simulink subsystem "Plant"  (R2022a)
settings: Solver=VariableStepAuto  StartTime=0.0  StopTime=10.0  RelTol=1e-3
settings Model: Creator=mmarq  LastModifiedBy=mmarq

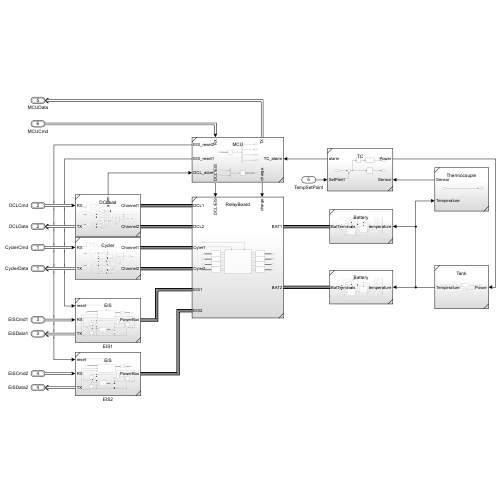
[thumbnail: Simulink's stored preview of the top-level diagram]
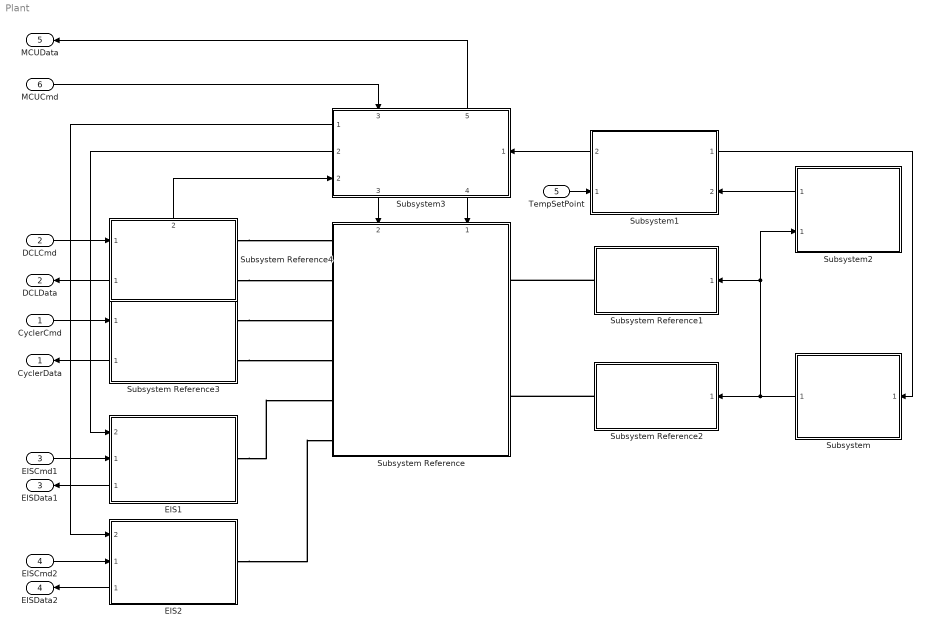
== system Plant ==
  CyclerCmd : Inport  OutputPortMessageModes=m  OutDataTypeStr=Bus: CyclerCmd  BusOutputAsStruct=on
  DCLCmd : Inport  OutputPortMessageModes=m  Port=2  OutDataTypeStr=Bus: DCLCmd  BusOutputAsStruct=on
  EISCmd1 : Inport  OutputPortMessageModes=m  Port=3  OutDataTypeStr=Bus: EISCmd  BusOutputAsStruct=on
  EISCmd2 : Inport  OutputPortMessageModes=m  Port=4  OutDataTypeStr=Bus: EISCmd  BusOutputAsStruct=on
  TempSetPoint : Inport  Port=5
  MCUCmd : Inport  OutputPortMessageModes=m  Port=6  OutDataTypeStr=Bus: MCUCmd  BusOutputAsStruct=on
  EIS1 : Subsystem  ReferencedSubsystem=EIS
      settings: PortSchema="{\"entries\":[{\"content\":{\"sides\":[{\"content\":{\"connectorIds\":[\"In2\",\"In1\",\"Out1\"]},\"type\":\"ConnectorPlacement.EquallySpacedRectSide\",\"uuid\":\"bda901de-5fc5-4df6-bed4-bf969933d972\"},{\"content\":{\"connectorIds\":[\"LConn1\"],\"side\":\"RIGHT\"},\"type\":\"ConnectorPlacement.EquallySpacedRectSide\",\"uuid\":\"97e6e5df-6a68-4cb9-aa40-ad9555eae5d3\"},{\"content\":{\"connectorIds\":[],\"side\":\"TOP\"},\"type\":\"ConnectorPlacement.EquallySpacedRectSide\",\"uuid\":\"3686a2fc-9119-406b-ac45-90d58aa6d823\"}]},\"type\":\"ConnectorPlacement.EquallySpacedConnector\",\"uuid\":\"6daecac9-5e0e-4dc6-b323-39bbe07465b3\"}],\"packageUris\":[\"http://schema.mathworks.com/mf0/Connector/R2020b\"],\"version\":\"1.0\"}"
  EIS2 : Subsystem  ReferencedSubsystem=EIS
      settings: PortSchema="{\"entries\":[{\"content\":{\"sides\":[{\"content\":{\"connectorIds\":[\"In2\",\"In1\",\"Out1\"]},\"type\":\"ConnectorPlacement.EquallySpacedRectSide\",\"uuid\":\"346fccca-2e03-4390-b8f8-dabc407f8e1d\"},{\"content\":{\"connectorIds\":[\"LConn1\"],\"side\":\"RIGHT\"},\"type\":\"ConnectorPlacement.EquallySpacedRectSide\",\"uuid\":\"347ef005-0f29-4770-89d9-3f34bb09e857\"},{\"content\":{\"connectorIds\":[],\"side\":\"TOP\"},\"type\":\"ConnectorPlacement.EquallySpacedRectSide\",\"uuid\":\"43d2187e-170b-4050-a904-0fbb5a542a24\"}]},\"type\":\"ConnectorPlacement.EquallySpacedConnector\",\"uuid\":\"0bc059c9-e074-4757-9a5e-e56a8190d977\"}],\"packageUris\":[\"http://schema.mathworks.com/mf0/Connector/R2020b\"],\"version\":\"1.0\"}"
  Subsystem : Subsystem  ReferencedSubsystem=Tank
  Subsystem Reference : Subsystem  ReferencedSubsystem=RelayBoard
      settings: PortSchema="{\"entries\":[{\"content\":{\"sides\":[{\"content\":{\"connectorIds\":[\"LConn3\",\"LConn7\",\"LConn2\",\"LConn6\",\"LConn4\",\"LConn8\"]},\"type\":\"ConnectorPlacement.EquallySpacedRectSide\",\"uuid\":\"2c82222c-b92b-4cb2-b168-0111504e6e71\"},{\"content\":{\"connectorIds\":[\"LConn1\",\"LConn5\"],\"side\":\"RIGHT\"},\"type\":\"ConnectorPlacement.EquallySpacedRectSide\",\"uuid\":\"59e2e9be-7ca9-4e66-8a31-f71f766dd2df\"},{\"content\":{\"connectorIds\":[\"In2\",\"In1\"],\"side\":\"TOP\"},\"type\":\"ConnectorPlacement.EquallySpacedRectSide\",\"uuid\":\"aebc3a48-61aa-4997-b1d8-73deb527f504\"}]},\"type\":\"ConnectorPlacement.EquallySpacedConnector\",\"uuid\":\"65ea92de-f703-4c73-ace1-0a27781508bc\"}],\"packageUris\":[\"http://schema.mathworks.com/mf0/Connector/R2020b\"],\"version\":\"1.0\"}"
  Subsystem Reference1 : Subsystem  ReferencedSubsystem=Battery
      settings: PortSchema="{\"entries\":[{\"content\":{\"sides\":[{\"content\":{\"connectorIds\":[\"LConn1\"]},\"type\":\"ConnectorPlacement.EquallySpacedRectSide\",\"uuid\":\"c15baa17-3528-45e3-b2fa-303e9d710e06\"},{\"content\":{\"connectorIds\":[\"In1\"],\"side\":\"RIGHT\"},\"type\":\"ConnectorPlacement.EquallySpacedRectSide\",\"uuid\":\"fb2fc25f-2319-470c-9cd2-01ed067f04f0\"},{\"content\":{\"connectorIds\":[],\"side\":\"TOP\"},\"type\":\"ConnectorPlacement.EquallySpacedRectSide\",\"uuid\":\"019a131c-ab68-4a32-933d-e5ce9d7fc5af\"}]},\"type\":\"ConnectorPlacement.EquallySpacedConnector\",\"uuid\":\"8ea13b11-84cd-4d75-b595-d58928f0c49e\"}],\"packageUris\":[\"http://schema.mathworks.com/mf0/Connector/R2020b\"],\"version\":\"1.0\"}"
  Subsystem Reference2 : Subsystem  ReferencedSubsystem=Battery
      settings: PortSchema="{\"entries\":[{\"content\":{\"sides\":[{\"content\":{\"connectorIds\":[\"LConn1\"]},\"type\":\"ConnectorPlacement.EquallySpacedRectSide\",\"uuid\":\"c15baa17-3528-45e3-b2fa-303e9d710e06\"},{\"content\":{\"connectorIds\":[\"In1\"],\"side\":\"RIGHT\"},\"type\":\"ConnectorPlacement.EquallySpacedRectSide\",\"uuid\":\"fb2fc25f-2319-470c-9cd2-01ed067f04f0\"},{\"content\":{\"connectorIds\":[],\"side\":\"TOP\"},\"type\":\"ConnectorPlacement.EquallySpacedRectSide\",\"uuid\":\"019a131c-ab68-4a32-933d-e5ce9d7fc5af\"}]},\"type\":\"ConnectorPlacement.EquallySpacedConnector\",\"uuid\":\"8ea13b11-84cd-4d75-b595-d58928f0c49e\"}],\"packageUris\":[\"http://schema.mathworks.com/mf0/Connector/R2020b\"],\"version\":\"1.0\"}"
  Subsystem Reference3 : Subsystem  ReferencedSubsystem=Cycler
      settings: PortSchema="{\"entries\":[{\"content\":{\"sides\":[{\"content\":{\"connectorIds\":[\"In1\",\"Out1\"]},\"type\":\"ConnectorPlacement.EquallySpacedRectSide\",\"uuid\":\"f71a85fa-5f1b-4f60-afc2-2af602cd6bfa\"},{\"content\":{\"connectorIds\":[\"LConn1\",\"LConn2\"],\"side\":\"RIGHT\"},\"type\":\"ConnectorPlacement.EquallySpacedRectSide\",\"uuid\":\"a58ae27e-7fda-4e3b-bf34-5bf7de7a0120\"},{\"content\":{\"connectorIds\":[],\"side\":\"TOP\"},\"type\":\"ConnectorPlacement.EquallySpacedRectSide\",\"uuid\":\"cf49a94a-a45d-4ba1-8d31-8fa348aa4236\"}]},\"type\":\"ConnectorPlacement.EquallySpacedConnector\",\"uuid\":\"5fb0b0ec-3310-4f5c-9c9c-9e0d49a0c2e5\"}],\"packageUris\":[\"http://schema.mathworks.com/mf0/Connector/R2020b\"],\"version\":\"1.0\"}"
  Subsystem Reference4 : Subsystem  ReferencedSubsystem=DCLoad
      settings: PortSchema="{\"entries\":[{\"content\":{\"sides\":[{\"content\":{\"connectorIds\":[\"In1\",\"Out1\"]},\"type\":\"ConnectorPlacement.EquallySpacedRectSide\",\"uuid\":\"f71a85fa-5f1b-4f60-afc2-2af602cd6bfa\"},{\"content\":{\"connectorIds\":[\"LConn1\",\"LConn2\"],\"side\":\"RIGHT\"},\"type\":\"ConnectorPlacement.EquallySpacedRectSide\",\"uuid\":\"a58ae27e-7fda-4e3b-bf34-5bf7de7a0120\"},{\"content\":{\"connectorIds\":[\"Out2\"],\"side\":\"TOP\"},\"type\":\"ConnectorPlacement.EquallySpacedRectSide\",\"uuid\":\"cf49a94a-a45d-4ba1-8d31-8fa348aa4236\"}]},\"type\":\"ConnectorPlacement.EquallySpacedConnector\",\"uuid\":\"5fb0b0ec-3310-4f5c-9c9c-9e0d49a0c2e5\"}],\"packageUris\":[\"http://schema.mathworks.com/mf0/Connector/R2020b\"],\"version\":\"1.0\"}"
  Subsystem1 : Subsystem  ReferencedSubsystem=TC
      settings: PortSchema="{\"entries\":[{\"content\":{\"sides\":[{\"content\":{\"connectorIds\":[\"Out2\",\"In1\"]},\"type\":\"ConnectorPlacement.EquallySpacedRectSide\",\"uuid\":\"9c6789b4-dd02-4592-85eb-f540f8ea46f0\"},{\"content\":{\"connectorIds\":[\"Out1\",\"In2\"],\"side\":\"RIGHT\"},\"type\":\"ConnectorPlacement.EquallySpacedRectSide\",\"uuid\":\"dd8c9bc9-ed02-469f-ae29-047c9d0545f6\"},{\"content\":{\"connectorIds\":[],\"side\":\"TOP\"},\"type\":\"ConnectorPlacement.EquallySpacedRectSide\",\"uuid\":\"0151dec0-87e3-4cf9-ba7c-3b720057dc11\"}]},\"type\":\"ConnectorPlacement.EquallySpacedConnector\",\"uuid\":\"b0e80b46-7a42-4e04-bf35-7b833283f7de\"}],\"packageUris\":[\"http://schema.mathworks.com/mf0/Connector/R2020b\"],\"version\":\"1.0\"}"
  Subsystem2 : Subsystem  ReferencedSubsystem=Thermocouple
      settings: PortSchema="{\"entries\":[{\"content\":{\"sides\":[{\"content\":{\"connectorIds\":[]},\"type\":\"ConnectorPlacement.EquallySpacedRectSide\",\"uuid\":\"0f8506b1-c558-4b53-9b84-b54b4f133099\"},{\"content\":{\"connectorIds\":[\"Out1\",\"In1\"],\"side\":\"RIGHT\"},\"type\":\"ConnectorPlacement.EquallySpacedRectSide\",\"uuid\":\"0c238bed-9bcf-499f-b949-06a843e9a6cc\"},{\"content\":{\"connectorIds\":[],\"side\":\"TOP\"},\"type\":\"ConnectorPlacement.EquallySpacedRectSide\",\"uuid\":\"4925469a-a1de-48f5-a3ee-e0cd87b78795\"}]},\"type\":\"ConnectorPlacement.EquallySpacedConnector\",\"uuid\":\"95810199-f4ed-42f7-878e-11f3bff63c1f\"}],\"packageUris\":[\"http://schema.mathworks.com/mf0/Connector/R2020b\"],\"version\":\"1.0\"}"
  Subsystem3 : Subsystem  ReferencedSubsystem=MCU
      settings: PortSchema="{\"entries\":[{\"content\":{\"sides\":[{\"content\":{\"connectorIds\":[\"Out1\",\"Out2\",\"In2\"]},\"type\":\"ConnectorPlacement.EquallySpacedRectSide\",\"uuid\":\"31e5b247-1279-4aa5-bbe4-47b63bcd243c\"},{\"content\":{\"connectorIds\":[\"In1\"],\"side\":\"RIGHT\"},\"type\":\"ConnectorPlacement.EquallySpacedRectSide\",\"uuid\":\"d31c3ffa-602f-4940-abd4-106385910974\"},{\"content\":{\"connectorIds\":[\"In3\",\"Out5\"],\"side\":\"TOP\"},\"type\":\"ConnectorPlacement.EquallySpacedRectSide\",\"uuid\":\"25b95ca8-96f9-4311-8680-e5e4fff5a408\"},{\"content\":{\"connectorIds\":[\"Out3\",\"Out4\"],\"side\":\"BOTTOM\"},\"type\":\"ConnectorPlacement.EquallySpacedRectSide\",\"uuid\":\"e024cf6d-8439-4201-b3f9-b92c54846c5e\"}]},\"type\":\"ConnectorPlacement.EquallySpacedConnector\",\"uuid\":\"3dda1080-8f2f-40dc-9e98-5ba3718b1061\"}],\"packageUris\":[\"http://schema.mathworks.com/mf0/Connector/R2020b\"],\"version\":\"1.0\"}"
  CyclerData : Outport  InputPortMessageModes=m  OutDataTypeStr=Bus: CyclerData  BusOutputAsStruct=on
  DCLData : Outport  InputPortMessageModes=m  Port=2  OutDataTypeStr=Bus: DCLData  BusOutputAsStruct=on
  EISData1 : Outport  InputPortMessageModes=m  Port=3  OutDataTypeStr=Bus: EISData  BusOutputAsStruct=on
  EISData2 : Outport  InputPortMessageModes=m  Port=4  OutDataTypeStr=Bus: EISData  BusOutputAsStruct=on
  MCUData : Outport  InputPortMessageModes=m  Port=5  OutDataTypeStr=Bus: MCUData  BusOutputAsStruct=on
  wires:
  EISCmd1/1 -> EIS1/1
  Subsystem3/2 -> EIS1/2
  Subsystem1/2 -> Subsystem3/1
  Subsystem3/1 -> EIS2/2
  Subsystem3/4 -> Subsystem Reference/1
  Subsystem1/1 -> Subsystem/1
  Subsystem/1 -> Subsystem Reference2/1, Subsystem2/1, Subsystem Reference1/1
  Subsystem2/1 -> Subsystem1/2
  Subsystem3/3 -> Subsystem Reference/2
  Subsystem3/5 -> MCUData/1
  EIS1/1 -> EISData1/1
  Subsystem Reference4/2 -> Subsystem3/2
  CyclerCmd/1 -> Subsystem Reference3/1
  DCLCmd/1 -> Subsystem Reference4/1
  EISCmd2/1 -> EIS2/1
  TempSetPoint/1 -> Subsystem1/1
  MCUCmd/1 -> Subsystem3/3
  Subsystem Reference4/1 -> DCLData/1
  EIS2/1 -> EISData2/1
  Subsystem Reference3/1 -> CyclerData/1
  connections:
  EIS1/LConn1 -- Subsystem Reference/LConn4
  Subsystem Reference2/LConn1 -- Subsystem Reference/LConn5
  Subsystem Reference1/LConn1 -- Subsystem Reference/LConn1
  EIS2/LConn1 -- Subsystem Reference/LConn8
  Subsystem Reference3/LConn1 -- Subsystem Reference/LConn2
  Subsystem Reference3/LConn2 -- Subsystem Reference/LConn6
  Subsystem Reference4/LConn2 -- Subsystem Reference/LConn7
  Subsystem Reference4/LConn1 -- Subsystem Reference/LConn3
